simulink library "cdsSWD1"  (Simulink 6.2)
settings Model: LastModifiedBy=rolf

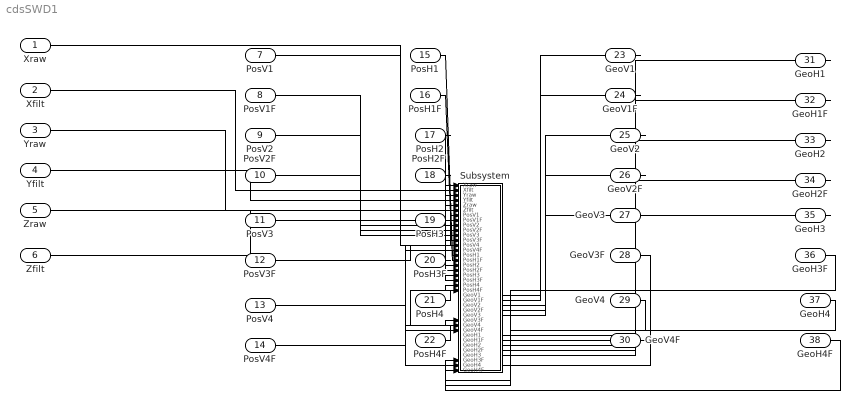
== system cdsSWD1 ==
  Xraw : Inport  Port=1  LatchInput=off
  Xfilt : Inport  Port=2  LatchInput=off
  Yraw : Inport  Port=3  LatchInput=off
  Yfilt : Inport  Port=4  LatchInput=off
  Zraw : Inport  Port=5  LatchInput=off
  Zfilt : Inport  Port=6  LatchInput=off
  PosV1 : Inport  Port=7  LatchInput=off
  PosV1F : Inport  Port=8  LatchInput=off
  PosV2 : Inport  Port=9  LatchInput=off
  PosV2F : Inport  Port=10  LatchInput=off
  PosV3 : Inport  Port=11  LatchInput=off
  PosV3F : Inport  Port=12  LatchInput=off
  PosV4 : Inport  Port=13  LatchInput=off
  PosV4F : Inport  Port=14  LatchInput=off
  PosH1 : Inport  Port=15  LatchInput=off
  PosH1F : Inport  Port=16  LatchInput=off
  PosH2 : Inport  Port=17  LatchInput=off
  PosH2F : Inport  Port=18  LatchInput=off
  PosH3 : Inport  Port=19  LatchInput=off
  PosH3F : Inport  Port=20  LatchInput=off
  PosH4 : Inport  Port=21  LatchInput=off
  PosH4F : Inport  Port=22  LatchInput=off
  GeoV1 : Inport  Port=23  LatchInput=off
  GeoV1F : Inport  Port=24  LatchInput=off
  GeoV2 : Inport  Port=25  LatchInput=off
  GeoV2F : Inport  Port=26  LatchInput=off
  GeoV3 : Inport  Port=27  LatchInput=off
  GeoV3F : Inport  Port=28  LatchInput=off
  GeoV4 : Inport  Port=29  LatchInput=off
  GeoV4F : Inport  Port=30  LatchInput=off
  GeoH1 : Inport  Port=31  LatchInput=off
  GeoH1F : Inport  Port=32  LatchInput=off
  GeoH2 : Inport  Port=33  LatchInput=off
  GeoH2F : Inport  Port=34  LatchInput=off
  GeoH3 : Inport  Port=35  LatchInput=off
  GeoH3F : Inport  Port=36  LatchInput=off
  GeoH4 : Inport  Port=37  LatchInput=off
  GeoH4F : Inport  Port=38  LatchInput=off
  Subsystem : Subsystem
  wires:
  Xraw/1 -> Subsystem/1(Xraw)
  Xfilt/1 -> Subsystem/2(Xfilt)
  Yraw/1 -> Subsystem/3(Yraw)
  Yfilt/1 -> Subsystem/4(Yfilt)
  Zraw/1 -> Subsystem/5(Zraw)
  Zfilt/1 -> Subsystem/6(Zfilt)
  PosV1/1 -> Subsystem/7(PosV1)
  PosV1F/1 -> Subsystem/8(PosV1F)
  PosV2/1 -> Subsystem/9(PosV2)
  PosV2F/1 -> Subsystem/10(PosV2F)
  PosV3/1 -> Subsystem/11(PosV3)
  PosV3F/1 -> Subsystem/12(PosV3F)
  PosV4/1 -> Subsystem/13(PosV4)
  PosV4F/1 -> Subsystem/14(PosV4F)
  PosH1/1 -> Subsystem/15(PosH1)
  PosH1F/1 -> Subsystem/16(PosH1F)
  PosH2/1 -> Subsystem/17(PosH2)
  PosH2F/1 -> Subsystem/18(PosH2F)
  PosH3/1 -> Subsystem/19(PosH3)
  PosH3F/1 -> Subsystem/20(PosH3F)
  PosH4/1 -> Subsystem/21(PosH4)
  PosH4F/1 -> Subsystem/22(PosH4F)
  GeoV1/1 -> Subsystem/23(GeoV1)
  GeoV1F/1 -> Subsystem/24(GeoV1F)
  GeoV2/1 -> Subsystem/25(GeoV2)
  GeoV2F/1 -> Subsystem/26(GeoV2F)
  GeoV3/1 -> Subsystem/27(GeoV3)
  GeoV3F/1 -> Subsystem/28(GeoV3F)
  GeoV4/1 -> Subsystem/29(GeoV4)
  GeoV4F/1 -> Subsystem/30(GeoV4F)
  GeoH1/1 -> Subsystem/31(GeoH1)
  GeoH1F/1 -> Subsystem/32(GeoH1F)
  GeoH2/1 -> Subsystem/33(GeoH2)
  GeoH2F/1 -> Subsystem/34(GeoH2F)
  GeoH3/1 -> Subsystem/35(GeoH3)
  GeoH3F/1 -> Subsystem/36(GeoH3F)
  GeoH4/1 -> Subsystem/37(GeoH4)
  GeoH4F/1 -> Subsystem/38(GeoH4F)

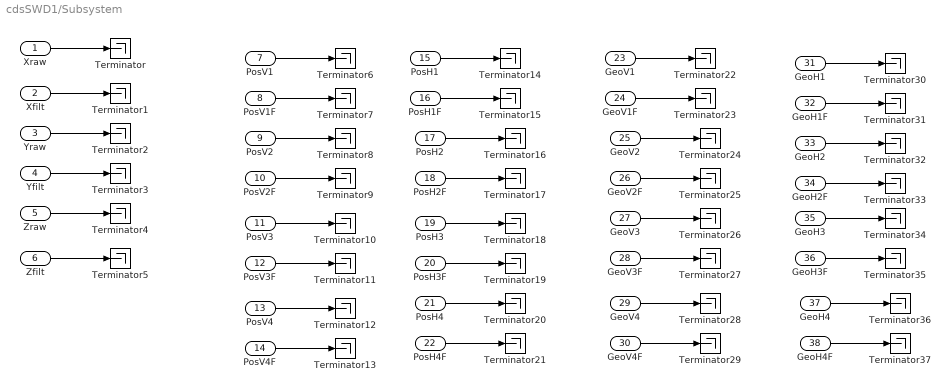
== system cdsSWD1/Subsystem ==
  Xraw : Inport  Port=1  LatchInput=off
  Xfilt : Inport  Port=2  LatchInput=off
  Yraw : Inport  Port=3  LatchInput=off
  Yfilt : Inport  Port=4  LatchInput=off
  Zraw : Inport  Port=5  LatchInput=off
  Zfilt : Inport  Port=6  LatchInput=off
  PosV1 : Inport  Port=7  LatchInput=off
  PosV1F : Inport  Port=8  LatchInput=off
  PosV2 : Inport  Port=9  LatchInput=off
  PosV2F : Inport  Port=10  LatchInput=off
  PosV3 : Inport  Port=11  LatchInput=off
  PosV3F : Inport  Port=12  LatchInput=off
  PosV4 : Inport  Port=13  LatchInput=off
  PosV4F : Inport  Port=14  LatchInput=off
  PosH1 : Inport  Port=15  LatchInput=off
  PosH1F : Inport  Port=16  LatchInput=off
  PosH2 : Inport  Port=17  LatchInput=off
  PosH2F : Inport  Port=18  LatchInput=off
  PosH3 : Inport  Port=19  LatchInput=off
  PosH3F : Inport  Port=20  LatchInput=off
  PosH4 : Inport  Port=21  LatchInput=off
  PosH4F : Inport  Port=22  LatchInput=off
  GeoV1 : Inport  Port=23  LatchInput=off
  GeoV1F : Inport  Port=24  LatchInput=off
  GeoV2 : Inport  Port=25  LatchInput=off
  GeoV2F : Inport  Port=26  LatchInput=off
  GeoV3 : Inport  Port=27  LatchInput=off
  GeoV3F : Inport  Port=28  LatchInput=off
  GeoV4 : Inport  Port=29  LatchInput=off
  GeoV4F : Inport  Port=30  LatchInput=off
  GeoH1 : Inport  Port=31  LatchInput=off
  GeoH1F : Inport  Port=32  LatchInput=off
  GeoH2 : Inport  Port=33  LatchInput=off
  GeoH2F : Inport  Port=34  LatchInput=off
  GeoH3 : Inport  Port=35  LatchInput=off
  GeoH3F : Inport  Port=36  LatchInput=off
  GeoH4 : Inport  Port=37  LatchInput=off
  GeoH4F : Inport  Port=38  LatchInput=off
  Terminator{,1..37} (38 alike) : Terminator
  wires:
  Xraw/1 -> Terminator/1
  Xfilt/1 -> Terminator1/1
  Yraw/1 -> Terminator2/1
  Yfilt/1 -> Terminator3/1
  Zraw/1 -> Terminator4/1
  Zfilt/1 -> Terminator5/1
  PosV1/1 -> Terminator6/1
  PosV1F/1 -> Terminator7/1
  PosV2/1 -> Terminator8/1
  PosV2F/1 -> Terminator9/1
  PosV3/1 -> Terminator10/1
  PosV3F/1 -> Terminator11/1
  PosV4/1 -> Terminator12/1
  PosV4F/1 -> Terminator13/1
  PosH1/1 -> Terminator14/1
  PosH1F/1 -> Terminator15/1
  PosH2/1 -> Terminator16/1
  PosH2F/1 -> Terminator17/1
  PosH3/1 -> Terminator18/1
  PosH3F/1 -> Terminator19/1
  PosH4/1 -> Terminator20/1
  PosH4F/1 -> Terminator21/1
  GeoV1/1 -> Terminator22/1
  GeoV1F/1 -> Terminator23/1
  GeoV2/1 -> Terminator24/1
  GeoV2F/1 -> Terminator25/1
  GeoV3/1 -> Terminator26/1
  GeoV3F/1 -> Terminator27/1
  GeoV4/1 -> Terminator28/1
  GeoV4F/1 -> Terminator29/1
  GeoH1/1 -> Terminator30/1
  GeoH1F/1 -> Terminator31/1
  GeoH2/1 -> Terminator32/1
  GeoH2F/1 -> Terminator33/1
  GeoH3/1 -> Terminator34/1
  GeoH3F/1 -> Terminator35/1
  GeoH4/1 -> Terminator36/1
  GeoH4F/1 -> Terminator37/1
